simulink model "quarter_car_pid_lqr_sim"  (R2023b)
settings: Solver=VariableStepAuto  StartTime=0.0  StopTime=60  RelTol=1e-3
values from neighbouring files (symbols this model uses):
  A = [0 1 0 0 ... (first row only)    [export_results.m]    (also in ga_lqr_tuning.m; main_ga_pid_lqr.m)
  B = [[0; -1/mus; 0; 1/mc], [0; kk/mus; 0; 0]]    [export_results.m]    (also in ga_lqr_tuning.m = [B1 B2]; main_ga_pid_lqr.m = [B1 B2])
  C = [0 0 1 0 ... (first row only)    [export_results.m]    (also in ga_lqr_tuning.m; main_ga_pid_lqr.m)
  Kd_base = K3_hat_base/(1+K3_hat_base*C*B)    [main_ga_pid_lqr.m]
  Kd_opt = K3_hat_opt/(1+K3_hat_opt*C*B)    [main_ga_pid_lqr.m]
  Ki_base = K1_hat_base*(1-Kd_base*C*B)    [main_ga_pid_lqr.m]
  Ki_opt = K1_hat_opt*(1-Kd_opt*C*B)    [main_ga_pid_lqr.m]
  Kp_base = K2_hat_base*(1-Kd_base*C*B)    [main_ga_pid_lqr.m]
  Kp_opt = K2_hat_opt*(1-Kd_opt*C*B)    [main_ga_pid_lqr.m]
settings Model: Creator=izmah  LastModifiedBy=izmah

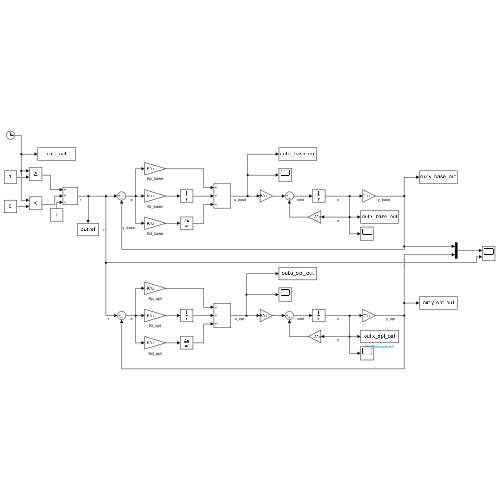
[thumbnail: Simulink's stored preview of the top-level diagram]
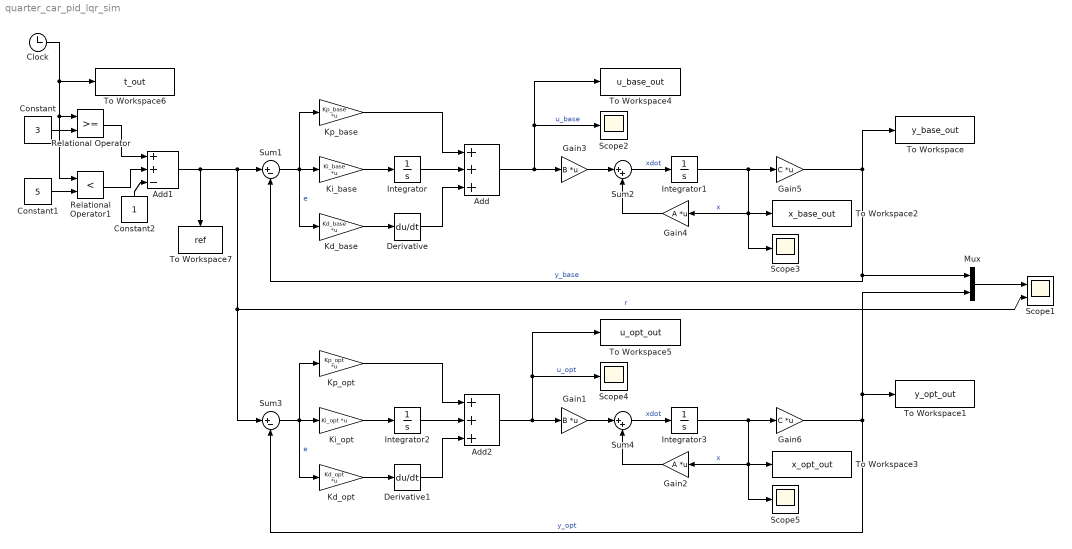
== system quarter_car_pid_lqr_sim ==
  Add : Sum  Inputs=+++
  Add1 : Sum  Inputs=++-
  Add2 : Sum  Inputs=+++
  Clock : Clock
  Constant : Constant  Value=3
  Constant1 : Constant  Value=5
  Constant2 : Constant
  Derivative : Derivative
  Derivative1 : Derivative
  Gain1 : Gain  Gain=B  Multiplication=Matrix(K*u)
  Gain2 : Gain  Gain=A  Multiplication=Matrix(K*u)
  Gain3 : Gain  Gain=B  Multiplication=Matrix(K*u)
  Gain4 : Gain  Gain=A  Multiplication=Matrix(K*u)
  Gain5 : Gain  Gain=C  Multiplication=Matrix(K*u)
  Gain6 : Gain  Gain=C  Multiplication=Matrix(K*u)
  Integrator{,1..3} (4 alike) : Integrator
  Kd_base : Gain  Gain=Kd_base  Multiplication=Matrix(K*u)
  Kd_opt : Gain  Gain=Kd_opt  Multiplication=Matrix(K*u)
  Ki_base : Gain  Gain=Ki_base  Multiplication=Matrix(K*u)
  Ki_opt : Gain  Gain=Ki_opt  Multiplication=Matrix(K*u)
  Kp_base : Gain  Gain=Kp_base  Multiplication=Matrix(K*u)
  Kp_opt : Gain  Gain=Kp_opt  Multiplication=Matrix(K*u)
  Mux : Mux  Inputs=2
  Relational Operator : RelationalOperator  OutDataTypeStr=boolean  RndMeth=Simplest  InputSameDT=off
  Relational Operator1 : RelationalOperator  Operator=<  OutDataTypeStr=boolean  RndMeth=Simplest  InputSameDT=off
  Scope1 : Scope  NumInputPorts=2
  Scope{2..5} (4 alike) : Scope
  Sum1 : Sum  Inputs=|+-
  Sum2 : Sum  Inputs=|++
  Sum3 : Sum  Inputs=|+-
  Sum4 : Sum  Inputs=|++
  To Workspace : ToWorkspace  VariableName=y_base_out  SampleTime=-1
  To Workspace1 : ToWorkspace  VariableName=y_opt_out  SampleTime=-1
  To Workspace2 : ToWorkspace  VariableName=x_base_out  SampleTime=-1
  To Workspace3 : ToWorkspace  VariableName=x_opt_out  SampleTime=-1
  To Workspace4 : ToWorkspace  VariableName=u_base_out  SampleTime=-1
  To Workspace5 : ToWorkspace  VariableName=u_opt_out  SampleTime=-1
  To Workspace6 : ToWorkspace  VariableName=t_out  SampleTime=-1
  To Workspace7 : ToWorkspace  VariableName=ref  SampleTime=-1
  wires:
  Sum2/1 -> Integrator1/1  "xdot"
  Gain3/1 -> Sum2/1
  Sum1/1 -> Ki_base/1, Kp_base/1, Kd_base/1  "e"
  Integrator1/1 -> To Workspace2/1, Scope3/1, Gain4/1, Gain5/1  "x"
  Gain5/1 -> Sum1/2, Mux/1, To Workspace/1  "y_base"
  Ki_base/1 -> Integrator/1
  Add/1 -> Gain3/1, Scope2/1, To Workspace4/1  "u_base"
  Gain4/1 -> Sum2/2
  Kd_base/1 -> Derivative/1
  Kp_base/1 -> Add/1
  Integrator/1 -> Add/2
  Derivative/1 -> Add/3
  Add1/1 -> Sum3/1, Scope1/2, Sum1/1, To Workspace7/1  "r"
  Relational Operator/1 -> Add1/1
  Constant2/1 -> Add1/3
  Relational Operator1/1 -> Add1/2
  Constant1/1 -> Relational Operator1/2
  Constant/1 -> Relational Operator/2
  Clock/1 -> Relational Operator/1, Relational Operator1/1, To Workspace6/1
  Sum3/1 -> Ki_opt/1, Kp_opt/1, Kd_opt/1  "e"
  Integrator2/1 -> Add2/2
  Add2/1 -> Scope4/1, To Workspace5/1, Gain1/1  "u_opt"
  Gain6/1 -> Mux/2, To Workspace1/1, Sum3/2  "y_opt"
  Sum4/1 -> Integrator3/1  "xdot"
  Gain2/1 -> Sum4/2
  Kp_opt/1 -> Add2/1
  Kd_opt/1 -> Derivative1/1
  Ki_opt/1 -> Integrator2/1
  Gain1/1 -> Sum4/1
  Derivative1/1 -> Add2/3
  Integrator3/1 -> To Workspace3/1, Scope5/1, Gain2/1, Gain6/1  "x"
  Mux/1 -> Scope1/1
